simulink model "Robust_RotPenFSFB"  (R2025b)
settings: Solver=VariableStepAuto  StartTime=0.0  StopTime=10  RelTol=1e-3
libraries: cstblocks x1
settings Model: Creator=djangovanderplas  LastModifiedBy=nstebbinsdahl

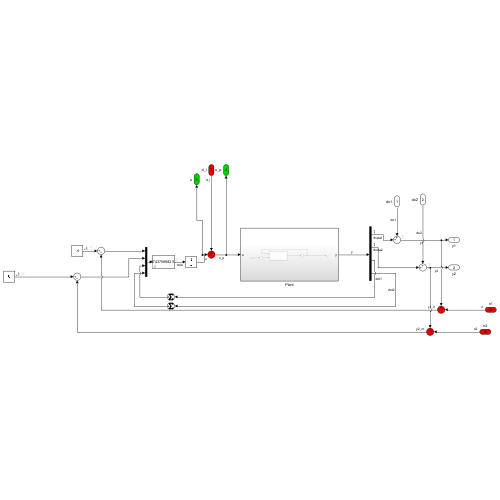
[thumbnail: Simulink's stored preview of the top-level diagram]
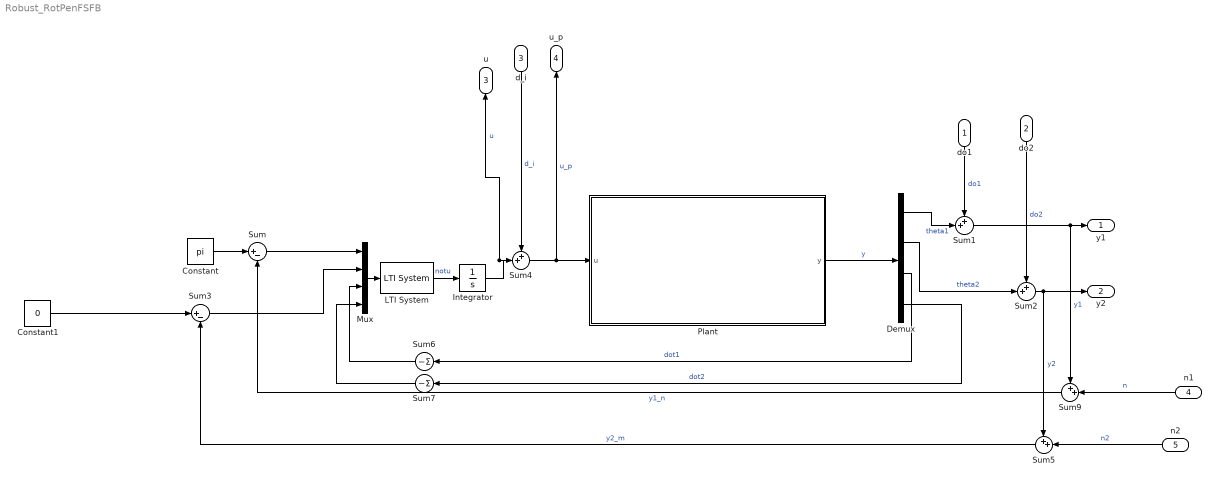
== system Robust_RotPenFSFB ==
  do1 : Inport  PortDimensions=1
  do2 : Inport  Port=2  PortDimensions=1
  d_i : Inport  Port=3
  n1 : Inport  Port=4  PortDimensions=1
  n2 : Inport  Port=5  PortDimensions=1
  Constant : Constant  Value=pi
  Constant1 : Constant  Value=0
  Demux : Demux
  Integrator : Integrator
  LTI System : cstblocks/LTI System  sys=ss([5.12294586858742 -1.33346087749101 0 0 0 0;11.6669672177865 -3.45315851065395 -0.105411748560781 0 0 0;0 -2.35706756203394 -9.29346877359186 -7.17996393969612 0 0;0 0 11.2781410931271 7.13092832886466 -2.184362728254 0;0 0 0 -0.211603596205927 -6.70051393489415 19.3535961197952;0 0 0 0 10.1617360843612 -69.596629608526],[6.72812315031749 -6.84066160622051 3.86292220201013 1.14891445128248;15.3241823706506 -15.4861840519365 8.69228857223768 0.478659327458437;8.56039743758982 5.78605602320375 0.133479829879575 -6.00649829679878;-14.9331327534141 1.67916795589068 -2.48200881795374 3.88968850542018;-0.539886462879739 1.30868681880876 5.78711931713972 9.08777529407953;5.45080850541922 4.10297923675778 -11.9716269944881 -35.5726645270393],[-0.233730984938798 0.629601444280092 0.0739796607503719 0.0349344179017065 -0.154057864165595 -0.0402957907661449],[9.7201539288621e-05 -9.7201539288621e-05 9.7201539288621e-05 -9.7201539288621e-05],0)  IC=[]  PadeOrder=0
  Mux : Mux
  Plant : Subsystem
  Sum : Sum  Inputs=|+-
  Sum{1..2,4..5,9} (5 alike) : Sum  Inputs=++|
  Sum3 : Sum  Inputs=|+-
  Sum6 : Sum  Inputs=-
  Sum7 : Sum  Inputs=-
  y1 : Outport  PortDimensions=1
  y2 : Outport  Port=2  PortDimensions=1
  u : Outport  Port=3
  u_p : Outport  Port=4
  wires:
  Plant/1(y) -> Demux/1  "y"
  Constant/1 -> Sum/1
  Demux/2 -> Sum2/2  "theta2"
  Demux/1 -> Sum1/2  "theta1"
  do1/1 -> Sum1/1  "do1"
  do2/1 -> Sum2/1  "do2"
  Sum1/1 -> y1/1, Sum9/1  "y1"
  Sum2/1 -> Sum5/1, y2/1  "y2"
  LTI System/1 -> Integrator/1  "notu"
  d_i/1 -> Sum4/1  "d_i"
  Sum4/1 -> Plant/1(u), u_p/1  "u_p"
  n1/1 -> Sum9/2  "n"
  n2/1 -> Sum5/2  "n2"
  Sum9/1 -> Sum/2  "y1_n"
  Sum5/1 -> Sum3/2  "y2_m"
  Constant1/1 -> Sum3/1
  Mux/1 -> LTI System/1
  Demux/3 -> Sum6/1  "dot1"
  Demux/4 -> Sum7/1  "dot2"
  Sum6/1 -> Mux/3
  Sum7/1 -> Mux/4
  Sum/1 -> Mux/1
  Sum3/1 -> Mux/2
  Integrator/1 -> u/1, Sum4/2  "u"

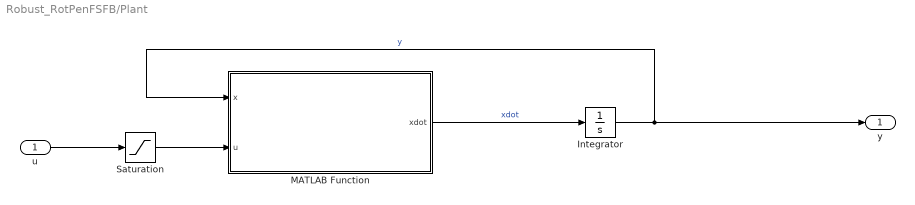
== system Robust_RotPenFSFB/Plant ==
  u : Inport
  Integrator : Integrator  InitialCondition=[pi+0.1;0.1;0.1;0.1]
  MATLAB Function : MATLAB Function  TreatAsAtomicUnit=on
  Saturation : Saturate  UpperLimit=1  LowerLimit=-1
  y : Outport
  wires:
  Integrator/1 -> y/1, MATLAB Function/1(x)  "y"
  MATLAB Function/1(xdot) -> Integrator/1  "xdot"
  u/1 -> Saturation/1
  Saturation/1 -> MATLAB Function/2(u)

== matlab function Robust_RotPenFSFB/Plant/MATLAB Function ==
  data: x input; u input; xdot output
function xdot = nonlinearPlant(x,u)

% State vector
theta1  = x(1);
theta2  = x(2);
dtheta1 = x(3);
dtheta2 = x(4);

% ============================================================
% Parameters
% ============================================================

pa       = 64.7915;
pb1      = 3.2117e3;
pc1      = 635.3865;
pg1      = 430.5226;
pu       = 2.2424e4;
p0       = 0;

pb2      = 0.0670;
pg2      = 112.0268;
pc2      = 0.2491;
psdelta2 = 0.1836;

epsv1    = 0.05;
epsv2    = 0.03;
vs2      = 3.5;

l1 = 0.1;
g  = 9.81;
pc = (l1/g)*pg2;

% ============================================================
% Dynamics
% ============================================================

c2 = cos(theta2);
s2 = sin(theta2);

% Inertia matrix
M11 = pa + 1 + 2*pc*c2;
M12 = 1 + pc*c2;
M21 = M12;
M22 = 1;

% Coriolis/Centrifugal terms
Cqdot1 = -pc*s2*(2*dtheta1*dtheta2 + dtheta2^2);
Cqdot2 =  pc*s2*dtheta1^2;

% Friction
F1 = pb1*dtheta1 + pc1*tanh(dtheta1/epsv1);

stribeck2 = pc2 + psdelta2*exp(-(dtheta2/vs2)^2);
F2 = pb2*dtheta2 + stribeck2*tanh(dtheta2/epsv2);

% Gravity
G1 = -pg1*sin(theta1) - pg2*sin(theta1 + theta2);
G2 = -pg2*sin(theta1 + theta2);

% Input torques
I1 = pu*u + p0;
I2 = 0;

% Right-hand side
rhs1 = I1 - Cqdot1 - F1 - G1;
rhs2 = I2 - Cqdot2 - F2 - G2;

% Solve M*qdd = rhs
detM = M11*M22 - M12*M21;

ddtheta1 = ( M22*rhs1 - M12*rhs2)/detM;
ddtheta2 = (-M21*rhs1 + M11*rhs2)/detM;

% State derivative
xdot = zeros(4,1);

xdot(1) = dtheta1;
xdot(2) = dtheta2;
xdot(3) = ddtheta1;
xdot(4) = ddtheta2;

end
